simulink model "Chapter_4_Section_3_Model"  (R2017a)
settings: Solver=ode4  StartTime=0.0  StopTime=200  FixedStep=stp_sz  MaxStep=.0001  MinStep=.00005  RelTol=1e-7  AbsTol=1e-7  EnableMultiTasking=on
InitFcn:
  | load Chapter_4_Section_3
  | warning off
StopFcn:
  | save data.mat u_simulation v_simulation psi_simulation r_simulation npr_user_provided npr_achievable alpha_user_provided alpha_achievable stp_sz
  | clear all
  | load('data.mat')
  | delete('data.mat')
values from neighbouring files (symbols this model uses):
  A_disk = 13.2025431267    [Chapter_4_Section_3.mat]
  a_r11 = [-0.000865667853776 -0.901318756108 0.00874486630837 -0.00765974060328 0.00955717632387 0.00641813989061 -0.011076069832 0.00201248118094 -0.00501952733262 0.00315605586996 -0.00210851076531 0.0148609220099 ... (324 elements, 18x18)]    [Chapter_4_Section_3.mat]
  a_r13 = [-0.0294995912119 -4.91037219533 -0.00332739568397 0.0888755061346 -0.00681796875441 0.183812407485 0.0112008036726 0.10429312155 -0.0251601482875 -0.228675692165 0.00453476042855 0.0594697753606 ... (169 elements, 13x13)]    [Chapter_4_Section_3.mat]
  a_r15 = [-0.00127786555898 0.776225741104 -0.00474776997752 -0.00131066749835 0.0137520402687 -0.00211384579247 8.8019955143e-05 -0.00028996241197 -0.00129826872567 -0.0202543144732 0.0030370404199 -0.00453425604591 ... (169 elements, 13x13)]    [Chapter_4_Section_3.mat]
  a_r22 = [-0.000797108949019 -1.01015556887 0.00406573750109 -0.00111578544774 0.00423859757219 -0.00799128279013 0.00569024815652 -0.0167562674532 0.00334935655618 -0.000712432292804 0.00154242142086 0.00240437743229 ... (169 elements, 13x13)]    [Chapter_4_Section_3.mat]
  a_r24 = [-0.000686927823555 -0.95665602689 0.00244839898375 0.00145613314595 -0.00607023426216 0.0163996841317 0.00152022458075 -0.000736874734971 -0.00294919321651 -0.000761800577268 -0.00251686123035 -0.00197732815976 ... (169 elements, 13x13)]    [Chapter_4_Section_3.mat]
  a_r26 = [-0.194397873228 1.89810259721 -0.0873186628061 -0.241231729519 0.281206161775 -0.16994038615 -0.116565511469 -0.0496572593209 0.0216084469732 0.0912933167406 0.0299797727001 0.0314987707028 ... (169 elements, 13x13)]    [Chapter_4_Section_3.mat]
  a_r31 = [-0.00489112559449 -3.89960530455 -0.0361162658575 0.0265931197764 0.0034376033088 0.000316401308368 -0.0243996243526 0.0792200139858 -0.023187698537 -0.0726743997029 0.00400632061963 -0.0350516560041 ... (169 elements, 13x13)]    [Chapter_4_Section_3.mat]
  a_r33 = [-0.601431448276 0.50360246711 0.500115950342 -0.0452293844892 -0.0181314142185 -0.0323524621531 0.0355826051968 0.0329239610677 0.0940919952313 0.0566642992805 -0.0379178935102 0.0254835488846 ... (169 elements, 13x13)]    [Chapter_4_Section_3.mat]
  a_r35 = [-0.861988746714 -0.582511154549 0.34264856173 -0.0655310417272 -0.417167685168 0.183176698588 -0.473887691644 -0.225677727522 -0.133571139717 -0.218168843707 0.0850592077583 -0.0257492082836 ... (169 elements, 13x13)]    [Chapter_4_Section_3.mat]
  a_r42 = [-0.000411079312172 -0.966350953459 0.00419936729713 0.00358740198521 -0.00356571428733 -0.00958951498266 -0.00230062261745 -3.48708248632e-05 -0.00350313209064 -0.00772126326768 -0.0011918234528 -0.00149424537901 ... (169 elements, 13x13)]    [Chapter_4_Section_3.mat]
  a_r44 = [-0.000156115728087 -0.944139704333 -0.00242185567679 0.00620214191605 0.00232565005277 -0.00625050722164 0.00126021167241 -0.000681873506535 0.0011931592381 -0.00289361611357 -0.00138182415247 -0.00252837386868 ... (169 elements, 13x13)]    [Chapter_4_Section_3.mat]
  a_r46 = [-0.000218462457517 1.89677852742 0.00896242354968 -0.00290259500747 0.00225128874867 0.00254539590487 0.00120681433209 0.00261900930035 0.00149629742842 0.000796832004109 0.00199591847947 0.00352664402036 ... (169 elements, 13x13)]    [Chapter_4_Section_3.mat]
  a_r51 = [-0.0010898880101 0.776080724329 0.000225388678941 0.00375234840616 -0.00838297691459 -0.00447310416982 -0.0119510882322 -0.00692765468718 0.00227273345413 -0.0063592610709 0.000914007544175 0.00943534814934 ... (169 elements, 13x13)]    [Chapter_4_Section_3.mat]
  a_r53 = [-0.83377539904 0.569677058563 0.434285019976 0.157205409215 -0.397195569542 -0.255164078245 -0.141246880777 0.177451291189 -0.182828550566 0.0648162508754 0.244251292681 0.160100487197 ... (169 elements, 13x13)]    [Chapter_4_Section_3.mat]
  a_r55 = [-0.000352406331634 0.764343029796 0.00339830320259 -0.000678251137483 -0.00243783779313 -0.00215979913278 0.00196909451093 -0.00577428819561 -0.00349811892924 -0.00488920883323 0.00112064970343 0.000774855197444 ... (169 elements, 13x13)]    [Chapter_4_Section_3.mat]
  a_r62 = [-0.546519039316 -1.22303009993 0.393735845548 -0.120016588191 0.38151861373 -0.213578592342 -0.602267954372 -0.105716444149 -0.153151371839 -0.163939447448 -0.555540353196 0.0685401630267 ... (169 elements, 13x13)]    [Chapter_4_Section_3.mat]
  a_r64 = [-0.0406191100017 -5.18251105957 -0.115497941507 -0.0935821370219 0.180972853448 -0.0201998949456 -0.0698170640352 -0.0736823539521 -0.034828919888 0.0876659960431 -0.0419335596239 -0.0240984963396 ... (169 elements, 13x13)]    [Chapter_4_Section_3.mat]
  a_r66 = [-0.00276803466684 1.11530008029 0.0229779449181 0.0262185319857 0.00628472844795 0.000156167369042 -0.00250093023805 -0.0114435042874 -0.00826774415326 -0.00991601759993 -0.00812142854996 0.0148245002111 ... (169 elements, 13x13)]    [Chapter_4_Section_3.mat]
  A_rudder = 6    [Chapter_4_Section_3.mat]
  alpha_max = 0.392699081699    [Chapter_4_Section_3.mat]
  b_r11 = [-1.91804272115 -67.7547902158 12.3212653748 -6.25011871643 13.082442224 5.48501776184 -10.1596546398 2.56004852009 -4.74360113798 3.95981895348 -2.02856412397 18.3264246889 ... (18 elements, 18x1)]    [Chapter_4_Section_3.mat]
  b_r13 = [9.68113335046 8.54720242819 0.883931047444 -5.56576078332 1.72641800243 -13.8756826027 -2.702777864 -9.4621991361 5.92943514782 22.6516835054 -1.0074598861 -6.31102592982 ... (13 elements, 13x1)]    [Chapter_4_Section_3.mat]
  b_r22 = [-8.230214728 -263.156134326 24.2327808151 -4.87921448873 19.1715641288 -45.8768653263 26.6325387064 -91.9399975548 16.6663243552 -3.80929112747 7.68030110892 12.8381492859 ... (13 elements, 13x1)]    [Chapter_4_Section_3.mat]
  b_r24 = [20.6689502907 674.321335078 -41.3637763247 -19.2444203625 82.0775505272 -259.897803047 -22.2545830602 11.3827604156 43.2189922355 11.7516897475 36.9394390446 30.4503929007 ... (13 elements, 13x1)]    [Chapter_4_Section_3.mat]
  b_r26 = [206.794755218 -62.242559329 24.5666904254 184.158146246 -103.419961827 115.160111337 76.4499795128 20.3457431208 -13.1704465249 -41.5730935141 -18.1334448714 -14.4641153742 ... (13 elements, 13x1)]    [Chapter_4_Section_3.mat]
  b_r31 = [3.76230189948 5.16928151238 2.64945725635 -18.4251953385 -2.0625905672 -0.18887543415 4.20433084471 -14.07893046 13.0563354882 16.4007691754 -2.13849071942 8.28528512456 ... (13 elements, 13x1)]    [Chapter_4_Section_3.mat]
  b_r33 = [-425.265727934 16.4952177922 163.76327445 -15.539902078 -6.59006558263 -11.1862310226 12.8543123126 11.4260264426 33.8206936715 19.7626944669 -13.5783728882 8.91023495161 ... (13 elements, 13x1)]    [Chapter_4_Section_3.mat]
  b_r35 = [955.467057384 23.8174564739 -126.402446683 48.3788727465 168.435579445 -128.161344325 216.24493699 142.979450788 65.1193355403 134.911935543 -50.7648858119 13.1799100865 ... (13 elements, 13x1)]    [Chapter_4_Section_3.mat]
  b_r42 = [15.9360311823 665.959154186 -98.5777560157 -55.5400651809 61.9220987195 200.312325561 47.5124103398 0.631683490985 64.1219861023 155.750535985 22.3985447876 29.803792586 ... (13 elements, 13x1)]    [Chapter_4_Section_3.mat]
  b_r44 = [-27.1891200017 -1761.50772747 -283.391471232 367.311489951 182.522124626 -579.755911925 104.353356772 -62.2376848714 99.3185259533 -260.784153955 -116.536414334 -226.454300618 ... (13 elements, 13x1)]    [Chapter_4_Section_3.mat]
  b_r46 = [-26.6906838426 431.487773123 657.709356633 -144.976364483 114.646575538 180.775978583 85.0953284375 135.592940904 78.9082960716 55.2973047721 106.740201988 241.432567993 ... (13 elements, 13x1)]    [Chapter_4_Section_3.mat]
  b_r51 = [-27.9768378982 741.05041888 2.33758926296 57.3995096963 -127.005620965 -47.2947833409 -133.876425682 -98.5907202753 26.0445243962 -88.3721242204 10.7680008324 130.122749963 ... (13 elements, 13x1)]    [Chapter_4_Section_3.mat]
  b_r53 = [949.455593416 -23.2452293814 -157.318364745 -121.412853107 173.067821874 177.10214052 64.7164189373 -120.452255472 86.0623964314 -43.0643550932 -116.39314584 -105.497696438 ... (13 elements, 13x1)]    [Chapter_4_Section_3.mat]
  b_r55 = [-217.127382907 9506.32343029 1148.82922273 -188.742556573 -694.43970838 -709.996440288 566.872400877 -1877.38940059 -1026.37679575 -1566.80129668 332.089563592 247.692614281 ... (13 elements, 13x1)]    [Chapter_4_Section_3.mat]
  b_r62 = [259.61149635 16.5485296799 -38.0095496792 45.1883806678 -40.3107166739 78.3455844965 73.5107367495 37.0054960802 51.6709447748 22.7410486275 84.4875008959 -21.9559289205 ... (13 elements, 13x1)]    [Chapter_4_Section_3.mat]
  b_r64 = [156.539833252 187.686482031 376.820920142 59.4312894666 -548.902692032 17.0176436095 70.7484878223 206.821047291 37.1716677759 -243.032149857 114.824775027 27.0037475025 ... (13 elements, 13x1)]    [Chapter_4_Section_3.mat]
  b_r66 = [-314.266256408 5285.46587095 1093.01941502 1627.30071258 387.633965073 8.0986510694 -130.443621448 -701.343286032 -436.49966457 -600.0481003 -433.735518303 884.367320612 ... (13 elements, 13x1)]    [Chapter_4_Section_3.mat]
  bettas_CQ = [0 5.39 17.77 34.97 50.79 58.7 64.55 68.33 73.49 85.2 93.11 102.75 ... (40 elements, 1x40)]    [Chapter_4_Section_3.mat]    (also in looking_up_n.m = [0 5.39 17.77 34.97 50.79 58.7 64.55 68.33 73.49 85.2 93.11 )
  bettas_CT = [0 5.37 16.73 33.6 44.63 60.82 73.22 80.46 86.3 92.15 100.41 110.74 ... (52 elements, 1x52)]    [Chapter_4_Section_3.mat]    (also in looking_up_n.m = [0 5.37 16.73 33.6 44.63 60.82 73.22 80.46 86.3 92.15 100.41)
  c_r11 = [1.91804272142 -67.7547902158 -12.3212653748 -6.25011871643 -13.082442224 5.48501776185 -10.1596546398 -2.56004852009 -4.74360113798 -3.95981895348 -2.02856412396 -18.3264246889 ... (18 elements, 1x18)]    [Chapter_4_Section_3.mat]
  c_r13 = [9.68113335045 -8.54720242824 0.883931047418 5.56576078332 1.72641800244 13.8756826027 -2.702777864 9.4621991361 5.92943514781 -22.6516835054 -1.0074598861 6.31102592982 ... (13 elements, 1x13)]    [Chapter_4_Section_3.mat]
  c_r22 = [8.23021472807 -263.156134326 -24.2327808151 -4.87921448871 19.1715641288 45.8768653263 26.6325387064 91.9399975548 16.6663243552 3.80929112749 7.68030110892 -12.8381492859 ... (13 elements, 1x13)]    [Chapter_4_Section_3.mat]
  c_r24 = [20.6689502903 -674.321335078 -41.3637763247 19.2444203625 -82.0775505271 -259.897803047 22.2545830602 11.3827604156 -43.2189922355 11.7516897475 -36.9394390446 30.4503929007 ... (13 elements, 1x13)]    [Chapter_4_Section_3.mat]
  c_r26 = [-206.794755218 -62.2425593289 24.5666904254 -184.158146246 -103.419961827 -115.160111337 -76.4499795128 20.3457431209 13.1704465249 -41.5730935141 18.1334448714 -14.4641153742 ... (13 elements, 1x13)]    [Chapter_4_Section_3.mat]
  c_r31 = [3.76230189951 -5.16928151238 -2.64945725636 -18.4251953385 -2.0625905672 -0.188875434257 -4.2043308447 14.07893046 13.0563354882 -16.4007691754 -2.13849071943 -8.28528512456 ... (13 elements, 1x13)]    [Chapter_4_Section_3.mat]
  c_r33 = [-425.265727934 -16.4952177923 -163.76327445 15.539902078 -6.5900655826 11.1862310226 12.8543123126 -11.4260264426 33.8206936715 -19.7626944669 -13.5783728882 -8.91023495161 ... (13 elements, 1x13)]    [Chapter_4_Section_3.mat]
  c_r35 = [-955.467057384 23.8174564746 -126.402446683 -48.3788727464 168.435579445 128.161344325 216.24493699 -142.979450788 65.1193355403 -134.911935543 50.7648858119 13.1799100865 ... (13 elements, 1x13)]    [Chapter_4_Section_3.mat]
  c_r42 = [15.9360311824 -665.959154186 -98.5777560157 55.5400651809 -61.9220987195 200.312325561 47.5124103398 -0.631683490192 -64.1219861023 155.750535985 -22.3985447876 29.803792586 ... (13 elements, 1x13)]    [Chapter_4_Section_3.mat]
  c_r44 = [27.189120009 -1761.50772747 283.391471232 367.311489951 182.522124626 579.755911925 104.353356772 62.2376848713 99.3185259533 260.784153955 -116.536414334 226.454300618 ... (13 elements, 1x13)]    [Chapter_4_Section_3.mat]
  c_r46 = [26.6906838375 431.487773123 -657.709356633 -144.976364484 114.646575538 -180.775978583 -85.0953284373 135.592940904 78.9082960717 -55.297304772 106.740201988 -241.432567993 ... (13 elements, 1x13)]    [Chapter_4_Section_3.mat]
  c_r51 = [27.9768378982 741.05041888 2.33758926325 -57.3995096963 127.005620965 -47.2947833409 -133.876425682 98.5907202753 26.0445243962 88.3721242204 10.7680008324 -130.122749963 ... (13 elements, 1x13)]    [Chapter_4_Section_3.mat]
  c_r53 = [-949.455593416 -23.2452293814 -157.318364745 121.412853107 173.067821874 -177.10214052 64.7164189374 120.452255472 86.0623964314 43.0643550932 -116.39314584 105.497696438 ... (13 elements, 1x13)]    [Chapter_4_Section_3.mat]
  c_r55 = [217.12738291 9506.32343029 -1148.82922273 -188.742556576 -694.43970838 709.996440288 566.872400876 1877.38940059 -1026.37679575 1566.80129668 332.089563594 -247.69261428 ... (13 elements, 1x13)]    [Chapter_4_Section_3.mat]
  c_r62 = [-259.61149635 16.5485296799 -38.0095496792 -45.1883806678 -40.3107166739 -78.3455844965 73.5107367495 -37.0054960802 -51.6709447748 22.7410486275 84.4875008959 21.9559289205 ... (13 elements, 1x13)]    [Chapter_4_Section_3.mat]
  c_r64 = [-156.539833251 187.686482031 -376.820920142 59.4312894666 548.902692032 17.0176436097 70.7484878223 -206.82104729 37.1716677758 243.032149857 -114.824775027 27.0037475025 ... (13 elements, 1x13)]    [Chapter_4_Section_3.mat]
  c_r66 = [314.266256408 5285.46587095 1093.01941502 -1627.30071258 -387.633965073 8.09865107118 -130.443621448 701.343286032 -436.49966457 600.0481003 -433.735518303 -884.367320612 ... (13 elements, 1x13)]    [Chapter_4_Section_3.mat]
  CQs = [0.008 0.007 -0.002 -0.018 -0.037 -0.049 -0.06 -0.065 -0.068 -0.059 -0.057 -0.059 ... (40 elements, 1x40)]    [Chapter_4_Section_3.mat]    (also in looking_up_n.m = -0.1.*[-0.08 -0.07 0.02 0.18 0.37 0.49 0.6 0.65 0.68 0.59 0.)
  CTs = [0.32 0.29 0.19 0.01 -0.16 -0.46 -0.7 -0.77 -0.7 -0.63 -0.63 -0.69 ... (52 elements, 1x52)]    [Chapter_4_Section_3.mat]    (also in looking_up_n.m = [0.32 0.29 0.19 0.01 -0.16 -0.46 -0.7 -0.77 -0.7 -0.63 -0.63)
  d_r11 = 95.5285227708    [Chapter_4_Section_3.mat]
  d_r13 = -14.1628545989    [Chapter_4_Section_3.mat]
  d_r22 = 1468.51041279    [Chapter_4_Section_3.mat]
  d_r24 = -9785.77027698    [Chapter_4_Section_3.mat]
  d_r26 = -1700.92421833    [Chapter_4_Section_3.mat]
  d_r31 = -0.95522945761    [Chapter_4_Section_3.mat]
  d_r33 = 3827.81220596    [Chapter_4_Section_3.mat]
  d_r35 = -19539.5268707    [Chapter_4_Section_3.mat]
  d_r42 = -9418.04264727    [Chapter_4_Section_3.mat]
  d_r44 = 68252.1479072    [Chapter_4_Section_3.mat]
  d_r46 = -10162.1377852    [Chapter_4_Section_3.mat]
  d_r51 = 12054.4514237    [Chapter_4_Section_3.mat]
  d_r53 = -19539.5038011    [Chapter_4_Section_3.mat]
  d_r55 = 1991036.95813    [Chapter_4_Section_3.mat]
  d_r62 = -1405.47636444    [Chapter_4_Section_3.mat]
  d_r64 = -12342.2523681    [Chapter_4_Section_3.mat]
  d_r66 = 610786.440495    [Chapter_4_Section_3.mat]
  DEN = 5.34671106464e+28    [Chapter_4_Section_3.mat]
  dist_LOS = [-50 -49 -48 -47 -46 -45 -44 -43 -42 -41 -40 -39 ... (1051 elements, 1x1051)]    [Chapter_4_Section_3.mat]
  Dpr = 4.1    [Chapter_4_Section_3.mat]    (also in looking_up_n.m = u(4))
  Dw = 0.110526315789    [Chapter_4_Section_3.mat]
  dx = 10    [Chapter_4_Section_3.mat]
  dxr = 48.75    [Chapter_4_Section_3.mat]
  dy = 2    [Chapter_4_Section_3.mat]
  dz = 0.8    [Chapter_4_Section_3.mat]
  dzr = 0.514285714286    [Chapter_4_Section_3.mat]
  g = 10    [Chapter_4_Section_3.mat]
  gravity = 10    [Chapter_4_Section_3.mat]
  INDEX = [1 2 3 4 5 6 7 8 9]    [Chapter_4_Section_3.mat]
  Ix = 724554000    [Chapter_4_Section_3.mat]
  Iy = 4528460000    [Chapter_4_Section_3.mat]
  Iz = 4528460000    [Chapter_4_Section_3.mat]
  k_wave = [0.0157865285852 0.0224311321394 0.0345394916241 0.0578593033576 0.0778685019714 0.0983501894009 0.10403521245 0.134043066308 0.155236404606 0.203205074918 0.220032771713 0.262178651673 ... (20 elements, 1x20)]    [Chapter_4_Section_3.mat]
  Last_Pt_Accuracy = 30    [Chapter_4_Section_3.mat]
  LBP = 100    [Chapter_4_Section_3.mat]
  m = 7264000    [Chapter_4_Section_3.mat]
  phase = [4.61787442739 6.09845039199 5.44708367148 0.54182753101 2.30238916367 2.31974450279 4.30416083443 3.75697809799 4.95971993271 2.31003141527 1.29451121971 0.54454197722 ... (20 elements, 1x20)]    [Chapter_4_Section_3.mat]
  phi_0 = 0    [Chapter_4_Section_3.mat]
  psi_0 = 0    [Chapter_4_Section_3.mat]
  R_convrg = 220    [Chapter_4_Section_3.mat]
  radius_LOS = [166.575605377 166.637026665 166.698699321 166.760625342 166.82280675 166.885245588 166.947943925 167.010903854 167.074127493 167.137616985 167.201374499 167.265402228 ... (1051 elements, 1x1051)]    [Chapter_4_Section_3.mat]
  raw = 1000    [Chapter_4_Section_3.mat]    (also in looking_up_n.m = u(3))
  s = 0.15    [Chapter_4_Section_3.mat]
  S11 = 5.22457985714e+28    [Chapter_4_Section_3.mat]
  S13 = 3.79917831589e+26    [Chapter_4_Section_3.mat]
  S15 = -4.97006200608e+19    [Chapter_4_Section_3.mat]
  S22 = 4.58630932583e+28    [Chapter_4_Section_3.mat]
  S24 = 9.38800137353e+19    [Chapter_4_Section_3.mat]
  S26 = 1.30387886946e+18    [Chapter_4_Section_3.mat]
  S31 = 3.83422033136e+26    [Chapter_4_Section_3.mat]
  S33 = 1.77296018417e+28    [Chapter_4_Section_3.mat]
  S35 = 2.44593333777e+19    [Chapter_4_Section_3.mat]
  S42 = 8.93369784557e+19    [Chapter_4_Section_3.mat]
  S44 = 7.37931315974e+19    [Chapter_4_Section_3.mat]
  S46 = 27990784014.6    [Chapter_4_Section_3.mat]
  S51 = -4.98658939538e+19    [Chapter_4_Section_3.mat]
  S53 = 2.45188465874e+19    [Chapter_4_Section_3.mat]
  S55 = 1.18069051188e+19    [Chapter_4_Section_3.mat]
  S62 = 1.30580221388e+18    [Chapter_4_Section_3.mat]
  S64 = 23535167243.9    [Chapter_4_Section_3.mat]
  S66 = 1.18069078235e+19    [Chapter_4_Section_3.mat]
  ... (+18 more)
undefined symbols (not defined in the file or in its folder): magnitude
libraries: simulink x9
(part 4 of 6)

== system Chapter_4_Section_3_Model/Ship_Model/Ship Dynamics with Environmental Forces and Memory Effect/Wave Excitation Force/wave elevation from multiple frequencies2/Seakeeping motion of the ship from RAO's and wave spectrum /Sea wave elevation from  ==
  w_star : Inport
  k_wave : Inport  Port=2
  phase : Inport  Port=3
  S : Inport  Port=4
  F_MOD : Inport  Port=5
  "F_PHASE " : Inport  Port=6
  X : Inport  Port=7
  Y : Inport  Port=8
  t : Inport  Port=9
  ksi : Inport  Port=10
  (sign convention for taw when z upwards,is multiplied by -1 for z downwards) : Gain  Gain=-1
  Gain : Gain  Gain=pi/180
  Math Function : Math  Operator=sqrt  SaturateOnIntegerOverflow=on
  Product{,2..4} (4 alike) : Product  RndMeth=Zero
  Product1 : Product  Inputs=3  RndMeth=Zero
  Product5 : Product  Inputs=3  RndMeth=Zero
  Read Me : simulink/Model-Wide Utilities/DocBlock  DocumentType=Text
  Sum : Sum  Inputs=|+|+|-|+
  Sum1 : Sum  Inputs=|+|+|
  Trigonometric Function : Trigonometry  Operator=cos
  Trigonometric Function1 : Trigonometry
  Trigonometric Function2 : Trigonometry  Operator=cos
  transforming Y to the z-upward -inertial frame(our inertial frame has z-downwards) : Gain  Gain=-1
  w12 : Constant  Value=2
  w13 : Constant  Value=Dw
  F : Outport
  wires:
  transforming Y to the z-upward -inertial frame(our inertial frame has z-downwards)/1 -> [Y]
  Product5/1 -> (sign convention for taw when z upwards,is multiplied by -1 for z downwards)/1
  Math Function/1 -> Product5/1
  Product1/1 -> Math Function/1
  [Dw] -> Product1/3
  [S] -> Product1/2
  w12/1 -> Product1/1
  Sum/1 -> Trigonometric Function2/1
  w13/1 -> [Dw]
  Product4/1 -> Sum/3
  [k_wave] -> Product4/1
  Sum1/1 -> Product4/2
  Product3/1 -> Sum1/2
  Product2/1 -> Sum1/1
  Trigonometric Function1/1 -> Product3/2
  [Y] -> Product3/1
  Trigonometric Function/1 -> Product2/2
  [X] -> Product2/1
  ksi/1 -> Trigonometric Function/1, Trigonometric Function1/1
  Y/1 -> transforming Y to the z-upward -inertial frame(our inertial frame has z-downwards)/1
  X/1 -> [X]
  phase/1 -> [phase]
  k_wave/1 -> [k_wave]
  w_star/1 -> [w_star]
  [phase] -> Sum/2
  Product/1 -> Sum/1
  [t] -> Product/2
  [w_star] -> Product/1
  t/1 -> [t]
  F_MOD/1 -> [F_MOD]
  "F_PHASE "/1 -> [F_PHASE]
  [F_PHASE] -> Gain/1
  Gain/1 -> Sum/4
  [F_MOD] -> Product5/2
  Trigonometric Function2/1 -> Product5/3
  (sign convention for taw when z upwards,is multiplied by -1 for z downwards)/1 -> F/1
  S/1 -> [S]
